simulink model "ES259A_BattVltgCorrln"  (R2013b)
settings: Solver=FixedStepDiscrete  SolverMode=SingleTasking  StartTime=0.0  StopTime=Inf  FixedStep=0.002  RelTol=1e-3
values from neighbouring files (symbols this model uses):
  BattVltgCorrlnAllwdVltgDif = DataDict.Calibration    [ES259A_BattVltgCorrln_DataDict.m]
  BattVltgCorrlnBattLoVltg = DataDict.Calibration    [ES259A_BattVltgCorrln_DataDict.m]
  BattVltgCorrlnBattOverVltg = DataDict.Calibration    [ES259A_BattVltgCorrln_DataDict.m]
  BattVltgCorrlnBattUnderVltg = DataDict.Calibration    [ES259A_BattVltgCorrln_DataDict.m]
  BattVltgCorrlnNtc0x03C0x0440x04CFailStep = DataDict.Calibration    [ES259A_BattVltgCorrln_DataDict.m]
  BattVltgCorrlnNtc0x03C0x0440x04CPassStep = DataDict.Calibration    [ES259A_BattVltgCorrln_DataDict.m]
  BattVltgCorrlnNtc0x03DFailStep = DataDict.Calibration    [ES259A_BattVltgCorrln_DataDict.m]
  BattVltgCorrlnNtc0x03DPassStep = DataDict.Calibration    [ES259A_BattVltgCorrln_DataDict.m]
  BattVltgCorrlnNtc0x0B0FailStep = DataDict.Calibration    [ES259A_BattVltgCorrln_DataDict.m]
  BattVltgCorrlnNtc0x0B0PassStep = DataDict.Calibration    [ES259A_BattVltgCorrln_DataDict.m]
  BattVltgCorrlnNtc0x0B1FailStep = DataDict.Calibration    [ES259A_BattVltgCorrln_DataDict.m]
  BattVltgCorrlnNtc0x0B1PassStep = DataDict.Calibration    [ES259A_BattVltgCorrln_DataDict.m]
  BattVltgCorrlnNtc0x0B5FailStep = DataDict.Calibration    [ES259A_BattVltgCorrln_DataDict.m]
  BattVltgCorrlnNtc0x0B5PassStep = DataDict.Calibration    [ES259A_BattVltgCorrln_DataDict.m]
  BattVltgCorrlnRcvrlBattLoVltg = DataDict.Calibration    [ES259A_BattVltgCorrln_DataDict.m]
  BattVltgCorrlnRcvrlBattOverVltg = DataDict.Calibration    [ES259A_BattVltgCorrln_DataDict.m]
  BattVltgCorrlnRcvrlBattUnderVltg = DataDict.Calibration    [ES259A_BattVltgCorrln_DataDict.m]
  BattVltgCorrlnSysMinVltg = DataDict.ImprtdCal    [ES250A_BattVltg_DataDict.m]    (also in ES259A_BattVltgCorrln_DataDict.m = DataDict.Calibration)
  BattVltgSwdMax = DataDict.Calibration    [ES250A_BattVltg_DataDict.m]
  ELECGLBPRM_STRTUPSTPWRDISCNCTBTESTCMPL_CNT_U08 = DataDict.Constant    [ES999A_ElecGlbPrm_DataDict.m]
  SYSVLTGFLTDUALIVTR_CNT_U08 = DataDict.Constant    [ES259A_BattVltgCorrln_DataDict.m]
undefined symbols (not defined in the file or in its folder): NtcNr1, NtcSts1, SigQlfr1
libraries: simulink x14
(part 5 of 7)

== system ES259A_BattVltgCorrln/BattVltgCorrln/BattVltgCorrlnPer1/WarmInit or Enable/Determine Independent Signals/Diagnose Inputs/NTC 3C/SetNtcSts 0x03C ==
  BattVltgOk : Inport
  Copyright1 : Subsystem  Description=|  mask(Copyright Information){none=on}
      | Copyright info block.                                               
      |                                                                     
      | Place copyright information at the top of every subsystem in design.
      mask prompts: none "No parameters"
      mask help: Place copyright information at the top of every subsystem in design.
      mask Display:
      | NxtrConf = 'Nexteer Confidential';
      | 
      | sys = bdroot; %handle for the current model ("system")
      | first = get_param(sys,'Created');
      | if(isempty(first))
      |     first = datestr(now,'yyyy');
      | else
      |     first = first(end-3:end);  %year is last four digits
      | end
      | 
      | last = get_param(sys,'LastModifiedDate');
      | if isempty(last)
      |     last = datestr(now,'yyyy');
      | else
      |     last = last(end-3:end);
      | end
      | 
      | if strcmp(first,last)
      |     fprintf('%s\nCopyright  %s Nexteer',NxtrConf,first);
      | else
      |     fprintf('%s\n%s%s-%s Nexteer',NxtrConf,char(169),first,last);
      | end
  Fails the test : Subsystem  RequirementInfo={} %GIDa_6ccae126_2072_4c7b_b3a0_362d219aba73  TreatAsAtomicUnit=on
  If : If  RequirementInfo={} %GIDa_793445dc_b67d_400c_8dd5_93229eed351d  IfExpression=u1 == 1
  Merge : Merge  RequirementInfo={} %GIDa_b447db53_c53b_43a2_8290_3641846b57ab
  Merge1 : Merge  RequirementInfo={} %GIDa_56ed8dd4_5c17_4ac1_846a_14dc68650043
  Merge2 : Merge  RequirementInfo={} %GIDa_f174f9cb_e878_44ec_99e2_09e0cfe3bff3
  Ntc Number (0x03C) : Constant  RequirementInfo={} %GIDa_0caafef0_b80a_4ba7_9183_596210a4b748  Value=NtcNr1.NTCNR_0X03C
  Passes the test : Subsystem  RequirementInfo={} %GIDa_466286b1_286b_453d_9eec_67f7012be75b  TreatAsAtomicUnit=on
  SetNtcSts : Subsystem  RequirementInfo={} %GIDa_bc20f90a_1006_45d5_bbf3_30fd97be1dc6
      settings: RTWSystemCode=Inline
  wires:
  BattVltgOk/1 -> If/1
  Merge2/1 -> SetNtcSts/4(DebStep)
  If/1 -> Passes the test/Action
  Passes the test/1(NtcInfo) -> Merge/1
  Passes the test/3(DebStep) -> Merge2/1
  Ntc Number (0x03C)/1 -> SetNtcSts/1(NtcNr)
  If/2 -> Fails the test/Action
  Fails the test/2(NtcSts) -> Merge1/2
  Merge1/1 -> SetNtcSts/3(NtcSts)
  Passes the test/2(NtcSts) -> Merge1/1
  Fails the test/1(NtcInfo) -> Merge/2
  Fails the test/3(DebStep) -> Merge2/2
  Merge/1 -> SetNtcSts/2(NtcStInfo)

== system ES259A_BattVltgCorrln/BattVltgCorrln/BattVltgCorrlnPer1/WarmInit or Enable/Determine Independent Signals/Diagnose Inputs/NTC 3D/Copyright1 ==

== system ES259A_BattVltgCorrln/BattVltgCorrln/BattVltgCorrlnPer1/WarmInit or Enable/Determine Independent Signals/Diagnose Inputs/NTC 3D/Fail NTC 3D ==
  Action Port : ActionPort  ActionType=then
  BattVltgCorrlnNtc0x03DFailStep : Constant  Value=BattVltgCorrlnNtc0x03DFailStep
  Copyright1 : Subsystem  Description=|  mask(Copyright Information){none=on}
      | Copyright info block.                                               
      |                                                                     
      | Place copyright information at the top of every subsystem in design.
      mask prompts: none "No parameters"
      mask help: Place copyright information at the top of every subsystem in design.
      mask Display:
      | NxtrConf = 'Nexteer Confidential';
      | 
      | sys = bdroot; %handle for the current model ("system")
      | first = get_param(sys,'Created');
      | if(isempty(first))
      |     first = datestr(now,'yyyy');
      | else
      |     first = first(end-3:end);  %year is last four digits
      | end
      | 
      | last = get_param(sys,'LastModifiedDate');
      | if isempty(last)
      |     last = datestr(now,'yyyy');
      | else
      |     last = last(end-3:end);
      | end
      | 
      | if strcmp(first,last)
      |     fprintf('%s\nCopyright  %s Nexteer',NxtrConf,first);
      | else
      |     fprintf('%s\n%s%s-%s Nexteer',NxtrConf,char(169),first,last);
      | end
  Ntc Number (0x03D) : Constant  RequirementInfo={} %GIDa_276f2b83_2a88_4016_911a_c57e2d67adef  Value=NtcNr1.NTCNR_0X03D
  Parameter Byte Data : Constant  Value=SYSVLTGFLTDUALIVTR_CNT_U08  VectorParams1D=off  OutDataTypeStr=uint8
  SetNtcSts : Subsystem  RequirementInfo={} %GIDa_135120b4_83bf_45b8_83ea_c9f4ae7772b3
      settings: RTWSystemCode=Inline
  Status Type : Constant  Value=NtcSts1.NTCSTS_PREFAILD
  wires:
  Ntc Number (0x03D)/1 -> SetNtcSts/1(NtcNr)
  Parameter Byte Data/1 -> SetNtcSts/2(NtcStInfo)
  Status Type/1 -> SetNtcSts/3(NtcSts)
  BattVltgCorrlnNtc0x03DFailStep/1 -> SetNtcSts/4(DebStep)

== system ES259A_BattVltgCorrln/BattVltgCorrln/BattVltgCorrlnPer1/WarmInit or Enable/Determine Independent Signals/Diagnose Inputs/NTC 3D/GetNtcQlfrSts ==
  note: Enumeration of SigQlfr1
      |         SIGQLFR_NORES   (0)
      |         SIGQLFR_PASSD    (1)
      |         SIGQLFR_FAILD      (2)
  NtcNr : Inport
  CopyRight2 : Subsystem  Description=|  mask(Copyright Information){none=on}
      | Copyright info block.                                               
      |                                                                     
      | Place copyright information at the top of every subsystem in design.
      mask prompts: none "No parameters"
      mask help: Place copyright information at the top of every subsystem in design.
      mask Display:
      | NxtrConf = 'Nexteer Confidential';
      | 
      | sys = bdroot; %handle for the current model ("system")
      | first = get_param(sys,'Created');
      | first = first(end-3:end);  %year is last four digits
      | 
      | last = get_param(sys,'LastModifiedDate');
      | if isempty(last)
      |     last = datestr(now,'yyyy');
      | else
      |     last = last(end-3:end);
      | end
      | 
      | if strcmp(first,last)
      |     fprintf('%s -- Copyright %s Nexteer',NxtrConf,first)
      | else
      |     fprintf('%s -- %s%s- %s Nexteer',NxtrConf,char(169),first,last)
      | end
  Data Store Read5 : DataStoreRead  DataStoreName=NtcQlfr3D
  Data Type Conversion : DataTypeConversion  OutDataTypeStr=uint8
  EOK : Constant  OutDataTypeStr=uint8
  Terminator : Terminator
  Return : Outport  InitialOutput=1
  Ntc0x03DQlfrSts : Outport  Port=2
  wires:
  Data Store Read5/1 -> Data Type Conversion/1
  EOK/1 -> Return/1
  NtcNr/1 -> Terminator/1
  Data Type Conversion/1 -> Ntc0x03DQlfrSts/1

== system ES259A_BattVltgCorrln/BattVltgCorrln/BattVltgCorrlnPer1/WarmInit or Enable/Determine Independent Signals/Diagnose Inputs/NTC 3D/Pass NTC 3D ==
  Action Port : ActionPort  ActionType=else
  BattVltgCorrlnNtc0x03DPassStep : Constant  Value=BattVltgCorrlnNtc0x03DPassStep  OutDataTypeStr=uint16
  Copyright1 : Subsystem  Description=|  mask(Copyright Information){none=on}
      | Copyright info block.                                               
      |                                                                     
      | Place copyright information at the top of every subsystem in design.
      mask prompts: none "No parameters"
      mask help: Place copyright information at the top of every subsystem in design.
      mask Display:
      | NxtrConf = 'Nexteer Confidential';
      | 
      | sys = bdroot; %handle for the current model ("system")
      | first = get_param(sys,'Created');
      | if(isempty(first))
      |     first = datestr(now,'yyyy');
      | else
      |     first = first(end-3:end);  %year is last four digits
      | end
      | 
      | last = get_param(sys,'LastModifiedDate');
      | if isempty(last)
      |     last = datestr(now,'yyyy');
      | else
      |     last = last(end-3:end);
      | end
      | 
      | if strcmp(first,last)
      |     fprintf('%s\nCopyright  %s Nexteer',NxtrConf,first);
      | else
      |     fprintf('%s\n%s%s-%s Nexteer',NxtrConf,char(169),first,last);
      | end
  Ntc Number (0x03D) : Constant  RequirementInfo={} %GIDa_6c72a04f_8062_44b2_9603_e047f206144a  Value=NtcNr1.NTCNR_0X03D
  Parameter Byte Data : Constant  Value=0  OutDataTypeStr=uint8
  SetNtcSts : Subsystem  RequirementInfo={} %GIDa_6b70d102_ed2b_4c18_9170_92f1b59f0041
      settings: RTWSystemCode=Inline
  Status Type : Constant  Value=NtcSts1.NTCSTS_PREPASSD  OutDataTypeStr=Enum: NtcSts1
  wires:
  Ntc Number (0x03D)/1 -> SetNtcSts/1(NtcNr)
  Parameter Byte Data/1 -> SetNtcSts/2(NtcStInfo)
  Status Type/1 -> SetNtcSts/3(NtcSts)
  BattVltgCorrlnNtc0x03DPassStep/1 -> SetNtcSts/4(DebStep)

== system ES259A_BattVltgCorrln/BattVltgCorrln/BattVltgCorrlnPer1/WarmInit or Enable/Determine Independent Signals/Diagnose Inputs/NTC 44/Copyright1 ==

== system ES259A_BattVltgCorrln/BattVltgCorrln/BattVltgCorrlnPer1/WarmInit or Enable/Determine Independent Signals/Diagnose Inputs/NTC 44/GetNtcQlfrSts 0x044 ==
  DiagcStsIvtr1Inactv : Inport
  Copyright1 : Subsystem  Description=|  mask(Copyright Information){none=on}
      | Copyright info block.                                               
      |                                                                     
      | Place copyright information at the top of every subsystem in design.
      mask prompts: none "No parameters"
      mask help: Place copyright information at the top of every subsystem in design.
      mask Display:
      | NxtrConf = 'Nexteer Confidential';
      | 
      | sys = bdroot; %handle for the current model ("system")
      | first = get_param(sys,'Created');
      | if(isempty(first))
      |     first = datestr(now,'yyyy');
      | else
      |     first = first(end-3:end);  %year is last four digits
      | end
      | 
      | last = get_param(sys,'LastModifiedDate');
      | if isempty(last)
      |     last = datestr(now,'yyyy');
      | else
      |     last = last(end-3:end);
      | end
      | 
      | if strcmp(first,last)
      |     fprintf('%s\nCopyright  %s Nexteer',NxtrConf,first);
      | else
      |     fprintf('%s\n%s%s-%s Nexteer',NxtrConf,char(169),first,last);
      | end
  Data Type Conversion : DataTypeConversion  OutDataTypeStr=uint8
  Data Type Conversion1 : DataTypeConversion  OutDataTypeStr=uint8
  GetNtcQlfrSts : Subsystem  RequirementInfo={} %GIDa_1d43ba10_2848_49bc_ac08_32c345cec887
  NTC 0x044 : Constant  RequirementInfo={} %GIDa_29918032_fa22_4534_8528_2fe7ad159701  Value=NtcNr1.NTCNR_0X044  OutDataTypeStr=Enum: NtcNr1
  NTC Fail Qlfr 0x044 : Constant  RequirementInfo={} %GIDa_ed54d07e_8a9d_40c8_a9a4_d750a3916030  Value=SigQlfr1.SIGQLFR_FAILD  OutDataTypeStr=Enum: SigQlfr1
  Return1 : Terminator
      settings: RequirementInfo={} %GIDa_7e3e9d96_5f15_4067_8f85_2e20bf70f2c8
  Switch : Switch  Criteria=u2 ~= 0
  Ntc0x044QlfrSts : Outport
  wires:
  NTC 0x044/1 -> GetNtcQlfrSts/1(NtcNr)
  GetNtcQlfrSts/1(Return) -> Return1/1
  DiagcStsIvtr1Inactv/1 -> Switch/2
  NTC Fail Qlfr 0x044/1 -> Data Type Conversion/1
  Switch/1 -> Ntc0x044QlfrSts/1
  Data Type Conversion/1 -> Switch/1
  Data Type Conversion1/1 -> Switch/3
  GetNtcQlfrSts/2(Ntc0x044QlfrSts) -> Data Type Conversion1/1

== system ES259A_BattVltgCorrln/BattVltgCorrln/BattVltgCorrlnPer1/WarmInit or Enable/Determine Independent Signals/Diagnose Inputs/NTC 44/SetNtcSts 0x044 ==
  BattVltgSwd1Ok : Inport  OutDataTypeStr=uint8
  DiagcStsIvtr1Inactv : Inport  RequirementInfo={} %GIDa_7b8bcc40_18bc_4378_ba26_0ace6bda9cd2  Port=2  OutDataTypeStr=boolean
  Copyright1 : Subsystem  Description=|  mask(Copyright Information){none=on}
      | Copyright info block.                                               
      |                                                                     
      | Place copyright information at the top of every subsystem in design.
      mask prompts: none "No parameters"
      mask help: Place copyright information at the top of every subsystem in design.
      mask Display:
      | NxtrConf = 'Nexteer Confidential';
      | 
      | sys = bdroot; %handle for the current model ("system")
      | first = get_param(sys,'Created');
      | if(isempty(first))
      |     first = datestr(now,'yyyy');
      | else
      |     first = first(end-3:end);  %year is last four digits
      | end
      | 
      | last = get_param(sys,'LastModifiedDate');
      | if isempty(last)
      |     last = datestr(now,'yyyy');
      | else
      |     last = last(end-3:end);
      | end
      | 
      | if strcmp(first,last)
      |     fprintf('%s\nCopyright  %s Nexteer',NxtrConf,first);
      | else
      |     fprintf('%s\n%s%s-%s Nexteer',NxtrConf,char(169),first,last);
      | end
  Do Nothing : Subsystem  RequirementInfo={} %GIDa_994a169a_c966_4350_8f4a_4790c77d0d03  TreatAsAtomicUnit=on
  Fails the test : Subsystem  RequirementInfo={} %GIDa_636d0796_118b_4b50_aa5a_96f8e7f6c289  TreatAsAtomicUnit=on
  For Simulation Only : DataTypeConversion  OutDataTypeStr=uint8
  If : If  RequirementInfo={} %GIDa_9233801e_fa77_4d5a_b854_52cbadc60e54  NumInputs=2  IfExpression=u2 == 1  ElseIfExpressions=u1 == 1
  Merge : Merge  RequirementInfo={} %GIDa_c45b7ce3_4438_47b7_a156_6d8f0bd22f82
  Merge1 : Merge  RequirementInfo={} %GIDa_c608d538_4a11_48a4_9013_338e53b7c25c
  Merge2 : Merge  RequirementInfo={} %GIDa_cfbe9729_58a5_44e9_9f7f_d3a1f2f9d3fc
  Ntc Number (0x044) : Constant  RequirementInfo={} %GIDa_74ee0374_a95f_430b_a97d_af6cf012a8d3  Value=NtcNr1.NTCNR_0X044
  Passes the test : Subsystem  RequirementInfo={} %GIDa_1ea0f243_8f50_480b_891c_edae25320667  TreatAsAtomicUnit=on
  SetNtcSts : Subsystem  RequirementInfo={} %GIDa_6fab68f7_0eff_4823_b0ed_d08d61603d18
      settings: RTWSystemCode=Inline
  wires:
  BattVltgSwd1Ok/1 -> If/1
  If/2 -> Passes the test/Action
  If/3 -> Fails the test/Action
  DiagcStsIvtr1Inactv/1 -> For Simulation Only/1
  If/1 -> Do Nothing/Action
  Ntc Number (0x044)/1 -> SetNtcSts/1(NtcNr)
  Passes the test/1(Ntc0x044 NtcStInfo) -> Merge/1
  Fails the test/1(Ntc0x044 NtcStInfo) -> Merge/2
  Passes the test/2(Ntc0x044 NtcSts) -> Merge1/1
  Fails the test/2(Ntc0x044 NtcSts) -> Merge1/2
  Passes the test/3(Ntc0x044 PassStep) -> Merge2/1
  Fails the test/3(Ntc0x044 FailStep) -> Merge2/2
  Merge/1 -> SetNtcSts/2(NtcStInfo)
  Merge1/1 -> SetNtcSts/3(NtcSts)
  Merge2/1 -> SetNtcSts/4(DebStep)
  For Simulation Only/1 -> If/2

== system ES259A_BattVltgCorrln/BattVltgCorrln/BattVltgCorrlnPer1/WarmInit or Enable/Determine Independent Signals/Diagnose Inputs/NTC 4C/Copyright1 ==

== system ES259A_BattVltgCorrln/BattVltgCorrln/BattVltgCorrlnPer1/WarmInit or Enable/Determine Independent Signals/Diagnose Inputs/NTC 4C/GetNtcQlfrSts 0x04C ==
  DiagcStsIvtr2Inactv : Inport
  Copyright1 : Subsystem  Description=|  mask(Copyright Information){none=on}
      | Copyright info block.                                               
      |                                                                     
      | Place copyright information at the top of every subsystem in design.
      mask prompts: none "No parameters"
      mask help: Place copyright information at the top of every subsystem in design.
      mask Display:
      | NxtrConf = 'Nexteer Confidential';
      | 
      | sys = bdroot; %handle for the current model ("system")
      | first = get_param(sys,'Created');
      | if(isempty(first))
      |     first = datestr(now,'yyyy');
      | else
      |     first = first(end-3:end);  %year is last four digits
      | end
      | 
      | last = get_param(sys,'LastModifiedDate');
      | if isempty(last)
      |     last = datestr(now,'yyyy');
      | else
      |     last = last(end-3:end);
      | end
      | 
      | if strcmp(first,last)
      |     fprintf('%s\nCopyright  %s Nexteer',NxtrConf,first);
      | else
      |     fprintf('%s\n%s%s-%s Nexteer',NxtrConf,char(169),first,last);
      | end
  Data Type Conversion2 : DataTypeConversion  OutDataTypeStr=uint8
  Data Type Conversion3 : DataTypeConversion  OutDataTypeStr=uint8
  GetNtcQlfrSts : Subsystem  RequirementInfo={} %GIDa_63523f19_fc83_4b2f_bc75_66bf8884b78f
  NTC 0x04C : Constant  RequirementInfo={} %GIDa_0152c6d4_fb57_406c_bedc_d3529fa81eb0  Value=NtcNr1.NTCNR_0X04C  OutDataTypeStr=Enum: NtcNr1
  NTC 0x04C1 : Constant  RequirementInfo={} %GIDa_e25d9d7b_c096_42d6_8dfd_ca27543c93fe  Value=SigQlfr1.SIGQLFR_FAILD  OutDataTypeStr=Enum: SigQlfr1  LockScale=on
  Return2 : Terminator
      settings: RequirementInfo={} %GIDa_c48a3c3b_58d1_4e1c_8841_2c40e79aed40
  Switch1 : Switch  Criteria=u2 ~= 0
  Ntc0x04CQlfrSts : Outport  OutDataTypeStr=uint8
  wires:
  NTC 0x04C/1 -> GetNtcQlfrSts/1(NtcNr)
  GetNtcQlfrSts/1(Return) -> Return2/1
  DiagcStsIvtr2Inactv/1 -> Switch1/2
  NTC 0x04C1/1 -> Data Type Conversion2/1
  Switch1/1 -> Ntc0x04CQlfrSts/1
  Data Type Conversion2/1 -> Switch1/1
  Data Type Conversion3/1 -> Switch1/3
  GetNtcQlfrSts/2(Ntc0x04CQlfrSts) -> Data Type Conversion3/1

== system ES259A_BattVltgCorrln/BattVltgCorrln/BattVltgCorrlnPer1/WarmInit or Enable/Determine Independent Signals/Diagnose Inputs/NTC 4C/SetNtcSts 0x04C ==
  BattVltgSwd2Ok : Inport  OutDataTypeStr=uint8
  DiagcStsIvtr2Inactv : Inport  RequirementInfo={} %GIDa_f0890c86_f27c_4565_90bb_930475e0efd1  Port=2  OutDataTypeStr=boolean
  Copyright1 : Subsystem  Description=|  mask(Copyright Information){none=on}
      | Copyright info block.                                               
      |                                                                     
      | Place copyright information at the top of every subsystem in design.
      mask prompts: none "No parameters"
      mask help: Place copyright information at the top of every subsystem in design.
      mask Display:
      | NxtrConf = 'Nexteer Confidential';
      | 
      | sys = bdroot; %handle for the current model ("system")
      | first = get_param(sys,'Created');
      | if(isempty(first))
      |     first = datestr(now,'yyyy');
      | else
      |     first = first(end-3:end);  %year is last four digits
      | end
      | 
      | last = get_param(sys,'LastModifiedDate');
      | if isempty(last)
      |     last = datestr(now,'yyyy');
      | else
      |     last = last(end-3:end);
      | end
      | 
      | if strcmp(first,last)
      |     fprintf('%s\nCopyright  %s Nexteer',NxtrConf,first);
      | else
      |     fprintf('%s\n%s%s-%s Nexteer',NxtrConf,char(169),first,last);
      | end
  Do Nothing : Subsystem  RequirementInfo={} %GIDa_1d593c9b_edee_4d9b_bfdd_966d85ed010b  TreatAsAtomicUnit=on
  Fails the test : Subsystem  RequirementInfo={} %GIDa_48143dc8_71bc_4c8c_b731_4c75cf818f49  TreatAsAtomicUnit=on
  For Simulation Only : DataTypeConversion  OutDataTypeStr=uint8
  If : If  RequirementInfo={} %GIDa_253ca524_57af_4167_a305_12926dc52cd5  NumInputs=2  IfExpression=u2 == 1  ElseIfExpressions=u1 == 1
  Merge : Merge  RequirementInfo={} %GIDa_2da756af_48a1_4e02_a9f7_817977a7553a
  Merge1 : Merge  RequirementInfo={} %GIDa_dc993944_6e77_4788_b12f_b5cb9bffa5ef
  Merge2 : Merge  RequirementInfo={} %GIDa_72ca6ae2_76e5_4ebe_9b7f_5e1be92309e8
  Ntc Number (0x04C) : Constant  RequirementInfo={} %GIDa_c269150d_0834_493a_ab40_d9382469fa96  Value=NtcNr1.NTCNR_0X04C
  Passes the test : Subsystem  RequirementInfo={} %GIDa_4abbea27_a889_4d10_8eba_9f69aac54360  TreatAsAtomicUnit=on
  SetNtcSts : Subsystem  RequirementInfo={} %GIDa_58558648_cfbd_422e_9b55_29c107b59528
      settings: RTWSystemCode=Inline
  wires:
  BattVltgSwd2Ok/1 -> If/1
  If/2 -> Passes the test/Action
  If/3 -> Fails the test/Action
  DiagcStsIvtr2Inactv/1 -> For Simulation Only/1
  If/1 -> Do Nothing/Action
  Merge/1 -> SetNtcSts/2(NtcStInfo)
  Merge1/1 -> SetNtcSts/3(NtcSts)
  Merge2/1 -> SetNtcSts/4(DebStep)
  Ntc Number (0x04C)/1 -> SetNtcSts/1(NtcNr)
  Passes the test/1(Ntc0x04C NtcStInfo) -> Merge/1
  Fails the test/1(Ntc0x04C NtcStInfo) -> Merge/2
  Passes the test/2(Ntc0x04C NtcSts) -> Merge1/1
  Fails the test/2(Ntc0x04C NtcSts) -> Merge1/2
  Passes the test/3(Ntc0x04C PassStep) -> Merge2/1
  Fails the test/3(Ntc0x04C PassStep) -> Merge2/2
  For Simulation Only/1 -> If/2

== system ES259A_BattVltgCorrln/BattVltgCorrln/BattVltgCorrlnPer1/WarmInit or Enable/Instantaneous Correlation/Correlation Check/BattVltg vs BattVltgSwd1/BattVltg <= 16 ==
  BattVltg : Inport  RequirementInfo={} %GIDa_2e73ff94_a90e_44aa_8aa6_33ffa26eb1a9
  BattVltgSwd1 : Inport  RequirementInfo={} %GIDa_69bca399_4ea3_4d84_b60e_9d185e791be8  Port=2
  BattVltgCorrlnAllwdVltgDif : Inport  RequirementInfo={} %GIDa_f6af9bf9_bfbf_43d8_932b_1f2401959bd3  Port=3
  Action Port : ActionPort  ActionType=then
  Abs2 : Abs  RequirementInfo={} %GIDa_76d1b796_3750_41ba_9bcc_4d7b4e0a0934  OutDataTypeStr=single
  Add1 : Sum  RequirementInfo={} %GIDa_2b44e491_2a93_4bb0_8979_ec6dc4807a22  Inputs=+-  AccumDataTypeStr=single
  Copyright1 : Subsystem  Description=|  RequirementInfo={} %GIDa_6ca8f19c_6789_4a74_b3fd_8d4392023beb  mask(Copyright Information){none=on}
      | Copyright info block.                                               
      |                                                                     
      | Place copyright information at the top of every subsystem in design.
      mask prompts: none "No parameters"
      mask help: Place copyright information at the top of every subsystem in design.
      mask Display:
      | NxtrConf = 'Nexteer Confidential';
      | 
      | sys = bdroot; %handle for the current model ("system")
      | first = get_param(sys,'Created');
      | if(isempty(first))
      |     first = datestr(now,'yyyy');
      | else
      |     first = first(end-3:end);  %year is last four digits
      | end
      | 
      | last = get_param(sys,'LastModifiedDate');
      | if isempty(last)
      |     last = datestr(now,'yyyy');
      | else
      |     last = last(end-3:end);
      | end
      | 
      | if strcmp(first,last)
      |     fprintf('%s\nCopyright  %s Nexteer',NxtrConf,first);
      | else
      |     fprintf('%s\n%s%s-%s Nexteer',NxtrConf,char(169),first,last);
      | end
  Relational Operator : RelationalOperator  RequirementInfo={} %GIDa_28ab3425_3e03_4f40_818a_52bd6540c8cd  Operator=<  OutDataTypeStr=boolean
  TestOk_Lgc : Outport  RequirementInfo={} %GIDa_915915b9_144d_49af_b383_051470ccbdc9
  wires:
  BattVltgSwd1/1 -> Add1/2
  Relational Operator/1 -> TestOk_Lgc/1
  BattVltgCorrlnAllwdVltgDif/1 -> Relational Operator/2
  BattVltg/1 -> Add1/1
  Add1/1 -> Abs2/1
  Abs2/1 -> Relational Operator/1

== system ES259A_BattVltgCorrln/BattVltgCorrln/BattVltgCorrlnPer1/WarmInit or Enable/Instantaneous Correlation/Correlation Check/BattVltg vs BattVltgSwd1/BattVltg > 16 ==
  BattVltgSwd1 : Inport  RequirementInfo={} %GIDa_049fae68_ca0d_4c4c_9477_1909cf4351c8
  BattVltgCorrlnAllwdVltgDif : Inport  RequirementInfo={} %GIDa_dd07736f_bec0_4fc7_a5bb_6e8e6a8b0dba  Port=2
  Action Port : ActionPort  ActionType=else
  Abs2 : Abs  RequirementInfo={} %GIDa_62118996_fbe8_49e7_83ae_ce82a6c56ac0  OutDataTypeStr=single
  Add1 : Sum  RequirementInfo={} %GIDa_c4e4ad03_af73_4e72_9c5d_ad3f1a9b00a9  Inputs=+-  AccumDataTypeStr=single
  Copyright1 : Subsystem  Description=|  RequirementInfo={} %GIDa_6554236f_9264_448f_807b_31c1496d9648  mask(Copyright Information){none=on}
      | Copyright info block.                                               
      |                                                                     
      | Place copyright information at the top of every subsystem in design.
      mask prompts: none "No parameters"
      mask help: Place copyright information at the top of every subsystem in design.
      mask Display:
      | NxtrConf = 'Nexteer Confidential';
      | 
      | sys = bdroot; %handle for the current model ("system")
      | first = get_param(sys,'Created');
      | if(isempty(first))
      |     first = datestr(now,'yyyy');
      | else
      |     first = first(end-3:end);  %year is last four digits
      | end
      | 
      | last = get_param(sys,'LastModifiedDate');
      | if isempty(last)
      |     last = datestr(now,'yyyy');
      | else
      |     last = last(end-3:end);
      | end
      | 
      | if strcmp(first,last)
      |     fprintf('%s\nCopyright  %s Nexteer',NxtrConf,first);
      | else
      |     fprintf('%s\n%s%s-%s Nexteer',NxtrConf,char(169),first,last);
      | end
  Maximum Switched Voltage : Constant  Value=BattVltgSwdMax
  Relational Operator : RelationalOperator  RequirementInfo={} %GIDa_2590ba0c_3bae_453e_bcf1_bc696d5f168f  Operator=<=  OutDataTypeStr=boolean
  TestOk_Lgc : Outport  RequirementInfo={} %GIDa_92b09e36_f17b_4baf_a0b7_fe6234438c4e
  wires:
  BattVltgCorrlnAllwdVltgDif/1 -> Relational Operator/2
  Relational Operator/1 -> TestOk_Lgc/1
  Maximum Switched Voltage/1 -> Add1/2
  BattVltgSwd1/1 -> Add1/1
  Add1/1 -> Abs2/1
  Abs2/1 -> Relational Operator/1

== system ES259A_BattVltgCorrln/BattVltgCorrln/BattVltgCorrlnPer1/WarmInit or Enable/Instantaneous Correlation/Correlation Check/BattVltg vs BattVltgSwd1/Copyright1 ==

== system ES259A_BattVltgCorrln/BattVltgCorrln/BattVltgCorrlnPer1/WarmInit or Enable/Instantaneous Correlation/Correlation Check/BattVltgSwd1 vs BattVltgSwd2/Copyright1 ==

== system ES259A_BattVltgCorrln/BattVltgCorrln/BattVltgCorrlnPer1/WarmInit or Enable/Instantaneous Correlation/Correlation Check/BattVltgSwd2 vs BattVltg/BattVltg <= 16 ==
  BattVltg : Inport  RequirementInfo={} %GIDa_f3eeb1cd_06ec_45a0_8a6e_9609a21b7b56
  BattVltgSwd2 : Inport  RequirementInfo={} %GIDa_110f2698_8749_4fd2_bd81_7189da540284  Port=2
  "BattVltgCorrlnAllwdVltgDif " : Inport  RequirementInfo={} %GIDa_b5927397_a0e2_445d_afea_9fcd5e02f5cb  Port=3
  Action Port : ActionPort  ActionType=then
  Abs2 : Abs  RequirementInfo={} %GIDa_9c03aab0_881a_4a8e_ab3d_83a7ab3e6da3  OutDataTypeStr=single
  Add1 : Sum  RequirementInfo={} %GIDa_f793bf07_979b_46c8_870a_faf9ceb0c6f8  Inputs=+-  AccumDataTypeStr=single
  Copyright1 : Subsystem  Description=|  RequirementInfo={} %GIDa_a89e0045_94bf_42ae_a15e_cee1e3b6fee6  mask(Copyright Information){none=on}
      | Copyright info block.                                               
      |                                                                     
      | Place copyright information at the top of every subsystem in design.
      mask prompts: none "No parameters"
      mask help: Place copyright information at the top of every subsystem in design.
      mask Display:
      | NxtrConf = 'Nexteer Confidential';
      | 
      | sys = bdroot; %handle for the current model ("system")
      | first = get_param(sys,'Created');
      | if(isempty(first))
      |     first = datestr(now,'yyyy');
      | else
      |     first = first(end-3:end);  %year is last four digits
      | end
      | 
      | last = get_param(sys,'LastModifiedDate');
      | if isempty(last)
      |     last = datestr(now,'yyyy');
      | else
      |     last = last(end-3:end);
      | end
      | 
      | if strcmp(first,last)
      |     fprintf('%s\nCopyright  %s Nexteer',NxtrConf,first);
      | else
      |     fprintf('%s\n%s%s-%s Nexteer',NxtrConf,char(169),first,last);
      | end
  Relational Operator : RelationalOperator  RequirementInfo={} %GIDa_b262b05f_79f6_4e03_bb47_8eaa4afc5339  Operator=<  OutDataTypeStr=boolean
  TestOk_Lgc : Outport  RequirementInfo={} %GIDa_b79ba34d_9658_44ae_b1ed_86a834ddb60d
  wires:
  BattVltgSwd2/1 -> Add1/2
  "BattVltgCorrlnAllwdVltgDif "/1 -> Relational Operator/2
  Add1/1 -> Abs2/1
  BattVltg/1 -> Add1/1
  Abs2/1 -> Relational Operator/1
  Relational Operator/1 -> TestOk_Lgc/1

== system ES259A_BattVltgCorrln/BattVltgCorrln/BattVltgCorrlnPer1/WarmInit or Enable/Instantaneous Correlation/Correlation Check/BattVltgSwd2 vs BattVltg/BattVltg > 16 ==
  BattVltgSwd2 : Inport  RequirementInfo={} %GIDa_e3b0ef47_f88c_42b2_bd46_6f83f85d73b2
  BattVltgCorrlnAllwdVltgDif : Inport  RequirementInfo={} %GIDa_bb2b2884_49e4_49e0_b718_d9820e687870  Port=2
  Action Port : ActionPort  ActionType=else
  Abs2 : Abs  RequirementInfo={} %GIDa_8a2f0dc9_64a9_4870_858a_b2a955714d8c  OutDataTypeStr=single
  Add : Sum  RequirementInfo={} %GIDa_80d700b5_97dc_4204_a49e_20d8de98b6ed  Inputs=+-  AccumDataTypeStr=single
  Copyright1 : Subsystem  Description=|  RequirementInfo={} %GIDa_08aee3b5_0099_4396_a3b4_1434a860e806  mask(Copyright Information){none=on}
      | Copyright info block.                                               
      |                                                                     
      | Place copyright information at the top of every subsystem in design.
      mask prompts: none "No parameters"
      mask help: Place copyright information at the top of every subsystem in design.
      mask Display:
      | NxtrConf = 'Nexteer Confidential';
      | 
      | sys = bdroot; %handle for the current model ("system")
      | first = get_param(sys,'Created');
      | if(isempty(first))
      |     first = datestr(now,'yyyy');
      | else
      |     first = first(end-3:end);  %year is last four digits
      | end
      | 
      | last = get_param(sys,'LastModifiedDate');
      | if isempty(last)
      |     last = datestr(now,'yyyy');
      | else
      |     last = last(end-3:end);
      | end
      | 
      | if strcmp(first,last)
      |     fprintf('%s\nCopyright  %s Nexteer',NxtrConf,first);
      | else
      |     fprintf('%s\n%s%s-%s Nexteer',NxtrConf,char(169),first,last);
      | end
  Maximum Switched Voltage : Constant  Value=BattVltgSwdMax
  Relational Operator : RelationalOperator  RequirementInfo={} %GIDa_0bbd40c2_f96b_4705_956d_4ccca65dba14  Operator=<=  OutDataTypeStr=boolean
  TestOk_Lgc : Outport  RequirementInfo={} %GIDa_89d25d02_d5b8_4c0a_879f_e511b862269c
  wires:
  BattVltgCorrlnAllwdVltgDif/1 -> Relational Operator/2
  Add/1 -> Abs2/1
  Relational Operator/1 -> TestOk_Lgc/1
  Maximum Switched Voltage/1 -> Add/2
  BattVltgSwd2/1 -> Add/1
  Abs2/1 -> Relational Operator/1

== system ES259A_BattVltgCorrln/BattVltgCorrln/BattVltgCorrlnPer1/WarmInit or Enable/Instantaneous Correlation/Correlation Check/BattVltgSwd2 vs BattVltg/Copyright1 ==

== system ES259A_BattVltgCorrln/BattVltgCorrln/BattVltgCorrlnPer1/WarmInit or Enable/Instantaneous Correlation/Correlation Check/DetermineSwitchedVoltageSaturated/Copyright1 ==

== system ES259A_BattVltgCorrln/BattVltgCorrln/BattVltgCorrlnPer1/WarmInit or Enable/Instantaneous Correlation/Range Check/BattVltgNotOk/Copyright1 ==

== system ES259A_BattVltgCorrln/BattVltgCorrln/BattVltgCorrlnPer1/WarmInit or Enable/Instantaneous Correlation/Range Check/BattVltgOk/Copyright1 ==

== system ES259A_BattVltgCorrln/BattVltgCorrln/BattVltgCorrlnPer1/WarmInit or Enable/Instantaneous Correlation/Range Check/BattVltgSwd1NotOk/Copyright1 ==

== system ES259A_BattVltgCorrln/BattVltgCorrln/BattVltgCorrlnPer1/WarmInit or Enable/Instantaneous Correlation/Range Check/BattVltgSwd1Ok/Copyright1 ==

== system ES259A_BattVltgCorrln/BattVltgCorrln/BattVltgCorrlnPer1/WarmInit or Enable/Instantaneous Correlation/Range Check/BattVltgSwd2NotOk/Copyright1 ==

== system ES259A_BattVltgCorrln/BattVltgCorrln/BattVltgCorrlnPer1/WarmInit or Enable/Instantaneous Correlation/Range Check/BattVltgSwd2Ok/Copyright1 ==

== system ES259A_BattVltgCorrln/BattVltgCorrln/BattVltgCorrlnPer1/Battery Voltage Diagnostics/Inhibition Off/LowVltg <= Batt <= OverVltg/If Action/SetNtcStsB0/Copyright1 ==

== system ES259A_BattVltgCorrln/BattVltgCorrln/BattVltgCorrlnPer1/Battery Voltage Diagnostics/Inhibition Off/LowVltg <= Batt <= OverVltg/If Action/SetNtcStsB5/Copyright1 ==

== system ES259A_BattVltgCorrln/BattVltgCorrln/BattVltgCorrlnPer1/Battery Voltage Diagnostics/Inhibition Off/LowVltg <= Batt <= OverVltg/If Action 1/SetNtcStsB0/Copyright1 ==

== system ES259A_BattVltgCorrln/BattVltgCorrln/BattVltgCorrlnPer1/Battery Voltage Diagnostics/Inhibition Off/LowVltg <= Batt <= OverVltg/If Action 1/SetNtcStsB1/Copyright1 ==

== system ES259A_BattVltgCorrln/BattVltgCorrln/BattVltgCorrlnPer1/Battery Voltage Diagnostics/Inhibition Off/LowVltg <= Batt <= OverVltg/No Fault Condition/SetNtcStsB0/Copyright1 ==

== system ES259A_BattVltgCorrln/BattVltgCorrln/BattVltgCorrlnPer1/Battery Voltage Diagnostics/Inhibition Off/LowVltg <= Batt <= OverVltg/No Fault Condition/SetNtcStsB1/Copyright1 ==

== system ES259A_BattVltgCorrln/BattVltgCorrln/BattVltgCorrlnPer1/Battery Voltage Diagnostics/Inhibition Off/LowVltg <= Batt <= OverVltg/No Fault Condition/SetNtcStsB5/Copyright1 ==

== system ES259A_BattVltgCorrln/BattVltgCorrln/BattVltgCorrlnPer1/Battery Voltage Diagnostics/Inhibition Off/UnderVltg <= BattVltg < LowVltg/If Action/SetNtcStsB1/Copyright1 ==

== system ES259A_BattVltgCorrln/BattVltgCorrln/BattVltgCorrlnPer1/Battery Voltage Diagnostics/Inhibition Off/UnderVltg <= BattVltg < LowVltg/If Action/SetNtcStsB5/Copyright1 ==

== system ES259A_BattVltgCorrln/BattVltgCorrln/BattVltgCorrlnPer1/Battery Voltage Diagnostics/Inhibition Off/UnderVltg <= BattVltg < LowVltg/If Action 1/SetNtcStsB0/Copyright1 ==

== system ES259A_BattVltgCorrln/BattVltgCorrln/BattVltgCorrlnPer1/Battery Voltage Diagnostics/Inhibition Off/UnderVltg <= BattVltg < LowVltg/If Action 1/SetNtcStsB1/Copyright1 ==

== system ES259A_BattVltgCorrln/BattVltgCorrln/BattVltgCorrlnPer1/Battery Voltage Diagnostics/Inhibition Off/UnderVltg <= BattVltg < LowVltg/If Action 1/SetNtcStsB5/Copyright1 ==

== system ES259A_BattVltgCorrln/BattVltgCorrln/BattVltgCorrlnPer1/WarmInit or Enable/Determine Independent Signals/Diagnose Inputs/NTC 3C/GetNtcQlfrSts /CopyRight2 ==

== system ES259A_BattVltgCorrln/BattVltgCorrln/BattVltgCorrlnPer1/WarmInit or Enable/Determine Independent Signals/Diagnose Inputs/NTC 3C/SetNtcSts 0x03C/Copyright1 ==

== system ES259A_BattVltgCorrln/BattVltgCorrln/BattVltgCorrlnPer1/WarmInit or Enable/Determine Independent Signals/Diagnose Inputs/NTC 3C/SetNtcSts 0x03C/Fails the test ==
  Action Port : ActionPort  ActionType=else
  BattVltgCorrlnNtc0x03CFailStep : Constant  Value=BattVltgCorrlnNtc0x03C0x0440x04CFailStep
  Copyright1 : Subsystem  Description=|  mask(Copyright Information){none=on}
      | Copyright info block.                                               
      |                                                                     
      | Place copyright information at the top of every subsystem in design.
      mask prompts: none "No parameters"
      mask help: Place copyright information at the top of every subsystem in design.
      mask Display:
      | NxtrConf = 'Nexteer Confidential';
      | 
      | sys = bdroot; %handle for the current model ("system")
      | first = get_param(sys,'Created');
      | if(isempty(first))
      |     first = datestr(now,'yyyy');
      | else
      |     first = first(end-3:end);  %year is last four digits
      | end
      | 
      | last = get_param(sys,'LastModifiedDate');
      | if isempty(last)
      |     last = datestr(now,'yyyy');
      | else
      |     last = last(end-3:end);
      | end
      | 
      | if strcmp(first,last)
      |     fprintf('%s\nCopyright  %s Nexteer',NxtrConf,first);
      | else
      |     fprintf('%s\n%s%s-%s Nexteer',NxtrConf,char(169),first,last);
      | end
  Parameter Byte : Constant  OutDataTypeStr=uint8
  Status Type : Constant  Value=NtcSts1.NTCSTS_PREFAILD
  NtcInfo : Outport  InitialOutput=1
  NtcSts : Outport  Port=2  InitialOutput=NtcSts1.NTCSTS_PREFAILD
  DebStep : Outport  Port=3  InitialOutput=BattVltgCorrlnNtc0x03C0x0440x04CFailStep
  wires:
  BattVltgCorrlnNtc0x03CFailStep/1 -> DebStep/1
  Status Type/1 -> NtcSts/1
  Parameter Byte/1 -> NtcInfo/1

== stateflow chart ES259A_BattVltgCorrln/BattVltgCorrln/BattVltgCorrlnPer1/Battery Voltage Diagnostics/Inhibition Off/LowVltg <= Batt <= OverVltg/If Action/SetNtcStsB5/ISO Fault Debounce Design NOT TO BE IMPLEMENTED IN THIS FDD USED ONLY FOR SIMULATION PURPOSES ==
  note: NTCSTS_PASSD           (0)
      | NTCSTS_FAILD             (1)
      | NTCSTS_PREPASSD   (2)
      | NTCSTS_PREFAILD     (3)
      |
      | SIGQLFR_NORES        (0)
      | SIGQLFR_PASSD         (1)
      | SIGQLFR_FAILD           (2)
  note: Fail step Loop
  note: Pass step Loop
  note: 
  (default) -> (junction 89)
  (junction 89) -> (junction 95) [order 1] : [NtcSts == 3]
  (junction 89) -> (junction 93) [order 2] : [ NtcSts == 2]
  (junction 93) -> (junction 230) [order 2] : {
      | DebCntr = DebCntr - DebStep;
      | }
  (junction 95) -> (junction 216) [order 2] : [DebCntr <= 0]
      | {
      | DebCntr = DebStep;
      | }
  (junction 95) -> (junction 103) [order 1] : [DebCntr > 0]
  (junction 93) -> (junction 123) [order 1] : [(DebCntr - DebStep) <= -32768]
      | {
      | DebCntr = -32768;
      | Qualifier = 1;
      | }
  (junction 230) -> (junction 231)
  (junction 103) -> (junction 216) [order 2] : {
      | DebCntr = DebCntr + DebStep;
      | }
  (junction 216) -> (junction 220) [order 2]
  (junction 216) -> (junction 220) [order 1] : [(DebCntr + DebStep) >=32767]
      | {
      | DebCntr = 32767;
      | Qualifier =2;
      | }
  (junction 103) -> (junction 220) [order 1] : [(DebCntr + DebStep) >=32767]
      | {
      | DebCntr = 32767;
      | Qualifier =2;
      | }
  (junction 220) -> (junction 141)
  (junction 123) -> (junction 141)
  (junction 231) -> (junction 123)
  (junction 141) -> (junction 159)
  data: NtcSts input uint8; Qualifier output uint8 =0; DebStep input uint16; DebCntr local int16

== stateflow chart ES259A_BattVltgCorrln/BattVltgCorrln/BattVltgCorrlnPer1/Battery Voltage Diagnostics/Inhibition Off/LowVltg <= Batt <= OverVltg/If Action 1/SetNtcStsB1/ISO Fault Debounce Design NOT TO BE IMPLEMENTED IN THIS FDD USED ONLY FOR SIMULATION PURPOSES ==
  note: NTCSTS_PASSD           (0)
      | NTCSTS_FAILD             (1)
      | NTCSTS_PREPASSD   (2)
      | NTCSTS_PREFAILD     (3)
      |
      | SIGQLFR_NORES        (0)
      | SIGQLFR_PASSD         (1)
      | SIGQLFR_FAILD           (2)
  note: Fail step Loop
  note: Pass step Loop
  note: 
  (default) -> (junction 89)
  (junction 89) -> (junction 95) [order 1] : [NtcSts == 3]
  (junction 89) -> (junction 93) [order 2] : [ NtcSts == 2]
  (junction 93) -> (junction 230) [order 2] : {
      | DebCntr = DebCntr - DebStep;
      | }
  (junction 95) -> (junction 216) [order 2] : [DebCntr <= 0]
      | {
      | DebCntr = DebStep;
      | }
  (junction 95) -> (junction 103) [order 1] : [DebCntr > 0]
  (junction 93) -> (junction 123) [order 1] : [(DebCntr - DebStep) <= -32768]
      | {
      | DebCntr = -32768;
      | Qualifier = 1;
      | }
  (junction 230) -> (junction 231)
  (junction 103) -> (junction 216) [order 2] : {
      | DebCntr = DebCntr + DebStep;
      | }
  (junction 216) -> (junction 220) [order 2]
  (junction 216) -> (junction 220) [order 1] : [(DebCntr + DebStep) >=32767]
      | {
      | DebCntr = 32767;
      | Qualifier =2;
      | }
  (junction 103) -> (junction 220) [order 1] : [(DebCntr + DebStep) >=32767]
      | {
      | DebCntr = 32767;
      | Qualifier =2;
      | }
  (junction 220) -> (junction 141)
  (junction 123) -> (junction 141)
  (junction 231) -> (junction 123)
  (junction 141) -> (junction 159)
  data: NtcSts input uint8; Qualifier output uint8 =0; DebStep input uint16; DebCntr local int16

== stateflow chart ES259A_BattVltgCorrln/BattVltgCorrln/BattVltgCorrlnPer1/Battery Voltage Diagnostics/Inhibition Off/LowVltg <= Batt <= OverVltg/No Fault Condition/SetNtcStsB5/ISO Fault Debounce Design NOT TO BE IMPLEMENTED IN THIS FDD USED ONLY FOR SIMULATION PURPOSES ==
  note: NTCSTS_PASSD           (0)
      | NTCSTS_FAILD             (1)
      | NTCSTS_PREPASSD   (2)
      | NTCSTS_PREFAILD     (3)
      |
      | SIGQLFR_NORES        (0)
      | SIGQLFR_PASSD         (1)
      | SIGQLFR_FAILD           (2)
  note: Fail step Loop
  note: Pass step Loop
  note: 
  (default) -> (junction 89)
  (junction 89) -> (junction 95) [order 1] : [NtcSts == 3]
  (junction 89) -> (junction 93) [order 2] : [ NtcSts == 2]
  (junction 93) -> (junction 230) [order 2] : {
      | DebCntr = DebCntr - DebStep;
      | }
  (junction 95) -> (junction 216) [order 2] : [DebCntr <= 0]
      | {
      | DebCntr = DebStep;
      | }
  (junction 95) -> (junction 103) [order 1] : [DebCntr > 0]
  (junction 93) -> (junction 123) [order 1] : [(DebCntr - DebStep) <= -32768]
      | {
      | DebCntr = -32768;
      | Qualifier = 1;
      | }
  (junction 230) -> (junction 231)
  (junction 103) -> (junction 216) [order 2] : {
      | DebCntr = DebCntr + DebStep;
      | }
  (junction 216) -> (junction 220) [order 2]
  (junction 216) -> (junction 220) [order 1] : [(DebCntr + DebStep) >=32767]
      | {
      | DebCntr = 32767;
      | Qualifier =2;
      | }
  (junction 103) -> (junction 220) [order 1] : [(DebCntr + DebStep) >=32767]
      | {
      | DebCntr = 32767;
      | Qualifier =2;
      | }
  (junction 220) -> (junction 141)
  (junction 123) -> (junction 141)
  (junction 231) -> (junction 123)
  (junction 141) -> (junction 159)
  data: NtcSts input uint8; Qualifier output uint8 =0; DebStep input uint16; DebCntr local int16

== system ES259A_BattVltgCorrln/BattVltgCorrln/BattVltgCorrlnPer1/WarmInit or Enable/Determine Independent Signals/Diagnose Inputs/NTC 3C/SetNtcSts 0x03C/Passes the test ==
  Action Port : ActionPort  ActionType=then
  BattVltgCorrlnNtc0x03CPassStep : Constant  Value=BattVltgCorrlnNtc0x03C0x0440x04CPassStep
  Copyright1 : Subsystem  Description=|  mask(Copyright Information){none=on}
      | Copyright info block.                                               
      |                                                                     
      | Place copyright information at the top of every subsystem in design.
      mask prompts: none "No parameters"
      mask help: Place copyright information at the top of every subsystem in design.
      mask Display:
      | NxtrConf = 'Nexteer Confidential';
      | 
      | sys = bdroot; %handle for the current model ("system")
      | first = get_param(sys,'Created');
      | if(isempty(first))
      |     first = datestr(now,'yyyy');
      | else
      |     first = first(end-3:end);  %year is last four digits
      | end
      | 
      | last = get_param(sys,'LastModifiedDate');
      | if isempty(last)
      |     last = datestr(now,'yyyy');
      | else
      |     last = last(end-3:end);
      | end
      | 
      | if strcmp(first,last)
      |     fprintf('%s\nCopyright  %s Nexteer',NxtrConf,first);
      | else
      |     fprintf('%s\n%s%s-%s Nexteer',NxtrConf,char(169),first,last);
      | end
  Parameter Byte Data1 : Constant  Value=0  OutDataTypeStr=uint8
  Status Type : Constant  Value=NtcSts1.NTCSTS_PREPASSD
  NtcInfo : Outport  InitialOutput=0
  NtcSts : Outport  Port=2  InitialOutput=NtcSts1.NTCSTS_PREPASSD
  DebStep : Outport  Port=3  InitialOutput=BattVltgCorrlnNtc0x03C0x0440x04CPassStep
  wires:
  BattVltgCorrlnNtc0x03CPassStep/1 -> DebStep/1
  Status Type/1 -> NtcSts/1
  Parameter Byte Data1/1 -> NtcInfo/1

== system ES259A_BattVltgCorrln/BattVltgCorrln/BattVltgCorrlnPer1/WarmInit or Enable/Determine Independent Signals/Diagnose Inputs/NTC 3C/SetNtcSts 0x03C/SetNtcSts ==
  note: Only pass values 2 or 3 as input to NtcSts.
      | 2: PrePassd
      | 3: PreFaild
  NtcNr : Inport
  NtcStInfo : Inport  Port=2
  NtcSts : Inport  Port=3
  DebStep : Inport  Port=4
  Copyright1 : Subsystem  Description=|  mask(Copyright Information){none=on}
      | Copyright info block.                                               
      |                                                                     
      | Place copyright information at the top of every subsystem in design.
      mask prompts: none "No parameters"
      mask help: Place copyright information at the top of every subsystem in design.
      mask Display:
      | NxtrConf = 'Nexteer Confidential';
      | 
      | sys = bdroot; %handle for the current model ("system")
      | first = get_param(sys,'Created');
      | if(isempty(first))
      |     first = datestr(now,'yyyy');
      | else
      |     first = first(end-3:end);  %year is last four digits
      | end
      | 
      | last = get_param(sys,'LastModifiedDate');
      | if isempty(last)
      |     last = datestr(now,'yyyy');
      | else
      |     last = last(end-3:end);
      | end
      | 
      | if strcmp(first,last)
      |     fprintf('%s\nCopyright  %s Nexteer',NxtrConf,first);
      | else
      |     fprintf('%s\n%s%s-%s Nexteer',NxtrConf,char(169),first,last);
      | end
  Data Store Write1 : DataStoreWrite  RequirementInfo={} %GIDa_53b068f0_1050_4667_9ad2_981ec6425be6  DataStoreName=NtcQlfr3C
  ISO Fault Debounce Design NOT TO BE IMPLEMENTED IN THIS FDD USED ONLY FOR SIMULATION PURPOSES : Stateflow chart  TreatAsAtomicUnit=on
  Only here because I could not get model to run with enumerations in the stateflow diagram : DataTypeConversion  OutDataTypeStr=uint8
  Terminator : Terminator
  Terminator1 : Terminator
  wires:
  NtcStInfo/1 -> Terminator1/1
  NtcNr/1 -> Terminator/1
  NtcSts/1 -> Only here because I could not get model to run with enumerations in the stateflow diagram/1
  DebStep/1 -> ISO Fault Debounce Design NOT TO BE IMPLEMENTED IN THIS FDD USED ONLY FOR SIMULATION PURPOSES/2(DebStep)
  Only here because I could not get model to run with enumerations in the stateflow diagram/1 -> ISO Fault Debounce Design NOT TO BE IMPLEMENTED IN THIS FDD USED ONLY FOR SIMULATION PURPOSES/1(NtcSts)
  ISO Fault Debounce Design NOT TO BE IMPLEMENTED IN THIS FDD USED ONLY FOR SIMULATION PURPOSES/1(Qualifier) -> Data Store Write1/1

== system ES259A_BattVltgCorrln/BattVltgCorrln/BattVltgCorrlnPer1/WarmInit or Enable/Determine Independent Signals/Diagnose Inputs/NTC 3D/Fail NTC 3D/Copyright1 ==

== system ES259A_BattVltgCorrln/BattVltgCorrln/BattVltgCorrlnPer1/WarmInit or Enable/Determine Independent Signals/Diagnose Inputs/NTC 3D/Fail NTC 3D/SetNtcSts ==
  note: Only pass values 2 or 3 as input to NtcSts.
      | 2: PrePassd
      | 3: PreFaild
  NtcNr : Inport
  NtcStInfo : Inport  Port=2
  NtcSts : Inport  Port=3
  DebStep : Inport  Port=4
  Copyright1 : Subsystem  Description=|  mask(Copyright Information){none=on}
      | Copyright info block.                                               
      |                                                                     
      | Place copyright information at the top of every subsystem in design.
      mask prompts: none "No parameters"
      mask help: Place copyright information at the top of every subsystem in design.
      mask Display:
      | NxtrConf = 'Nexteer Confidential';
      | 
      | sys = bdroot; %handle for the current model ("system")
      | first = get_param(sys,'Created');
      | if(isempty(first))
      |     first = datestr(now,'yyyy');
      | else
      |     first = first(end-3:end);  %year is last four digits
      | end
      | 
      | last = get_param(sys,'LastModifiedDate');
      | if isempty(last)
      |     last = datestr(now,'yyyy');
      | else
      |     last = last(end-3:end);
      | end
      | 
      | if strcmp(first,last)
      |     fprintf('%s\nCopyright  %s Nexteer',NxtrConf,first);
      | else
      |     fprintf('%s\n%s%s-%s Nexteer',NxtrConf,char(169),first,last);
      | end
  Data Store Write1 : DataStoreWrite  RequirementInfo={} %GIDa_bc717a8d_8c5b_491f_9600_e784f8d55a86  DataStoreName=NtcQlfr3D
  ISO Fault Debounce Design NOT TO BE IMPLEMENTED IN THIS FDD USED ONLY FOR SIMULATION PURPOSES : Stateflow chart  TreatAsAtomicUnit=on
  Only here because I could not get model to run with enumerations in the stateflow diagram : DataTypeConversion  OutDataTypeStr=uint8
  Terminator : Terminator
  Terminator1 : Terminator
  wires:
  NtcStInfo/1 -> Terminator1/1
  NtcNr/1 -> Terminator/1
  NtcSts/1 -> Only here because I could not get model to run with enumerations in the stateflow diagram/1
  DebStep/1 -> ISO Fault Debounce Design NOT TO BE IMPLEMENTED IN THIS FDD USED ONLY FOR SIMULATION PURPOSES/2(DebStep)
  ISO Fault Debounce Design NOT TO BE IMPLEMENTED IN THIS FDD USED ONLY FOR SIMULATION PURPOSES/1(Qualifier) -> Data Store Write1/1
  Only here because I could not get model to run with enumerations in the stateflow diagram/1 -> ISO Fault Debounce Design NOT TO BE IMPLEMENTED IN THIS FDD USED ONLY FOR SIMULATION PURPOSES/1(NtcSts)

== system ES259A_BattVltgCorrln/BattVltgCorrln/BattVltgCorrlnPer1/WarmInit or Enable/Determine Independent Signals/Diagnose Inputs/NTC 3D/GetNtcQlfrSts/CopyRight2 ==
